simulink model "sin_input"  (R2021b)
settings: Solver=FixedStepAuto  StartTime=0.0  StopTime=10.0  RelTol=1e-3  EnableMultiTasking=on
libraries: arduinolib x4
settings Model: ExtModeTrigDuration=2  Creator=Erfan  LastModifiedBy=Erfan
settings OptimizationCC: EnhancedBackFolding=on  PassReuseOutputArgsAs=Individual arguments  ZeroExternalMemoryAtStartup=off  ZeroInternalMemoryAtStartup=off  MaxStackSize=64  OptimizeBlockOrder=speed  DifferentSizesBufferReuse=on  OptimizationCustomize=off  EfficientTunableParamExpr=on
settings DebuggingCC: ParameterTunabilityLossMsg=error
settings HardwareCC: ProdBitPerPointer=32  ProdBitPerSizeT=32  ProdBitPerPtrDiffT=32  ProdLargestAtomicInteger=Long  ProdLargestAtomicFloat=Double  ProdWordSize=32  ProdHWDeviceType=ARM Compatible->ARM Cortex
settings SFSimCC: MATLABDynamicMemAlloc=off
settings RTWCC: Description=Embedded Coder  SystemTargetFile=ert.tlc  HardwareBoard=Arduino Due  TemplateMakefile=ert_default_tmf  Toolchain=Arduino ARM  BuildConfiguration=Faster Runs
settings CodeAppCC: ForceParamTrailComments=on  IgnoreCustomStorageClasses=off  OperatorAnnotations=on  SimulinkDataObjDesc=on  SFDataObjDesc=on  InsertBlockDesc=on
settings ERTTargetCC: SupportContinuousTime=on  SupportVariableSizeSignals=on  ExtModeTransport=3  ExtModeStaticAlloc=on  ExtModeStaticAllocSize=24576  ExtModeMexFile=ext_xcp  ExtModeIntrfLevel=Level2 - Open

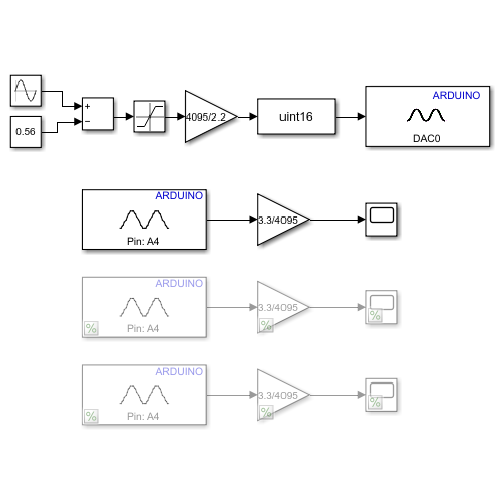
[thumbnail: Simulink's stored preview of the top-level diagram]
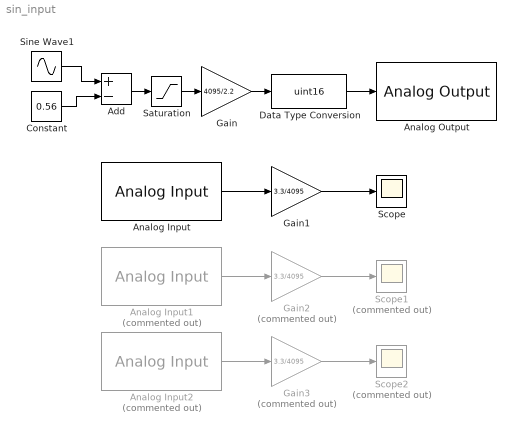
== system sin_input ==
  Add : Sum  Inputs=+-
  Analog Input : arduinolib/Analog Input  pinNumber=4  ReadResultsOnly=off  ConversionTriggerSource=Software  ExternalTriggerType=uint32( 0 )  OutputDataType=uint16  EnableConversionCompleteNotify=off  EnableOuputStatus=off  SampleTime=0.1  blockPlatform=arduino
  Analog Input1 : arduinolib/Analog Input  Commented=on  pinNumber=4  ReadResultsOnly=off  ConversionTriggerSource=Software  ExternalTriggerType=uint32( 0 )  OutputDataType=uint16  EnableConversionCompleteNotify=off  EnableOuputStatus=off  SampleTime=0.5  blockPlatform=arduino
  Analog Input2 : arduinolib/Analog Input  Commented=on  pinNumber=4  ReadResultsOnly=off  ConversionTriggerSource=Software  ExternalTriggerType=uint32( 0 )  OutputDataType=uint16  EnableConversionCompleteNotify=off  EnableOuputStatus=off  SampleTime=0.01  blockPlatform=arduino
  Analog Output : arduinolib/Analog Output  DACpin=DAC0  blockPlatform=arduino
      settings: SourceProductBaseCode=ARDUINO
  Constant : Constant  Value=0.56
  Data Type Conversion : DataTypeConversion  OutDataTypeStr=uint16
  Gain : Gain  Gain=4095/2.2
  Gain1 : Gain  Gain=3.3/4095
  Gain2 : Gain  Commented=on  Gain=3.3/4095
  Gain3 : Gain  Commented=on  Gain=3.3/4095
  Saturation : Saturate  UpperLimit=2.2  LowerLimit=0
  Scope : Scope
  Scope1 : Scope  Commented=on
  Scope2 : Scope  Commented=on
  Sine Wave1 : Sin  Bias=1.5  SampleTime=0
  wires:
  Gain1/1 -> Scope/1
  Analog Input/1 -> Gain1/1
  Add/1 -> Saturation/1
  Data Type Conversion/1 -> Analog Output/1
  Saturation/1 -> Gain/1
  Gain/1 -> Data Type Conversion/1
  Constant/1 -> Add/2
  Sine Wave1/1 -> Add/1
  Analog Input1/1 -> Gain2/1
  Gain2/1 -> Scope1/1
  Gain3/1 -> Scope2/1
  Analog Input2/1 -> Gain3/1
